simulink model "sim_validate_rint"  (Simulink 3.00)
settings: Solver=ode1  StartTime=starttime  StopTime=endtime  FixedStep=.5  RelTol=1e-3
values from neighbouring files (symbols this model uses):
  pwr_data = -1*pwr_data    [validate_rc.m]    (also in validate_rc_results.m = pwr_data(1:endi); validate_rc_results_2models.m = pwr_data(1:endi))
  t_data = t_data-t_data(1)    [validate_rc.m]    (also in validate_rc_results.m = t_data(1:endi); validate_rc_results_2models.m = t_data(1:endi))
libraries: lib_energy_storage x1
settings Model: LastModifiedBy=vjohnson

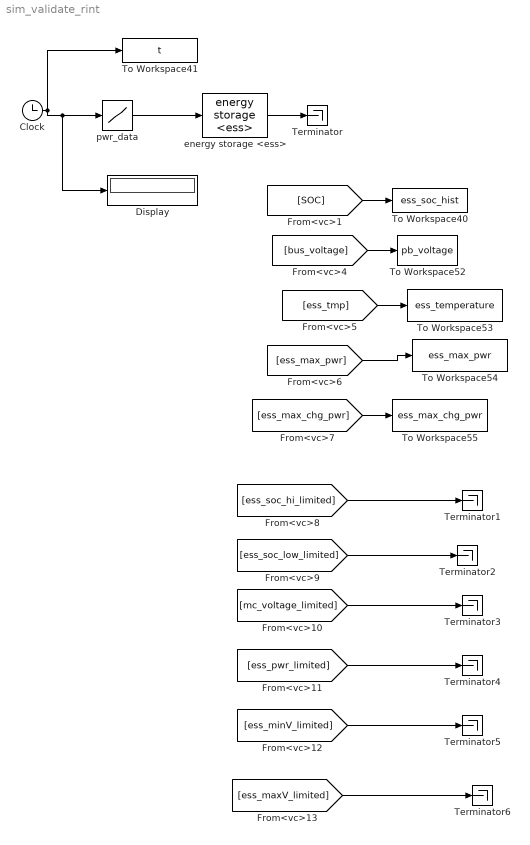
== system sim_validate_rint ==
  Clock : Clock
      settings: DisplayTime=off  Decimation=10
  Display : Display
      settings: Format=short
  Terminator{,1..6} (7 alike) : Terminator
  To Workspace40 : ToWorkspace  VariableName=ess_soc_hist  SampleTime=-1  SaveFormat=Matrix
  To Workspace41 : ToWorkspace  VariableName=t  SampleTime=-1  SaveFormat=Matrix
  To Workspace52 : ToWorkspace  VariableName=pb_voltage  SampleTime=-1  SaveFormat=Matrix
  To Workspace53 : ToWorkspace  VariableName=ess_temperature  SampleTime=-1  SaveFormat=Matrix
  To Workspace54 : ToWorkspace  VariableName=ess_max_pwr  SampleTime=-1  SaveFormat=Matrix
  To Workspace55 : ToWorkspace  VariableName=ess_max_chg_pwr  SampleTime=-1  SaveFormat=Matrix
  energy storage <ess> : lib_energy_storage/energy storage <ess>
  pwr_data : Lookup  InputValues=t_data  OutputValues=pwr_data
  wires:
  pwr_data/1 -> energy storage <ess>/1
  energy storage <ess>/1 -> Terminator/1
  [bus_voltage] -> To Workspace52/1
  [SOC] -> To Workspace40/1
  [ess_tmp] -> To Workspace53/1
  [ess_max_pwr] -> To Workspace54/1
  [ess_max_chg_pwr] -> To Workspace55/1
  Clock/1 -> To Workspace41/1, pwr_data/1, Display/1
  [ess_soc_hi_limited] -> Terminator1/1
  [ess_soc_low_limited] -> Terminator2/1
  [mc_voltage_limited] -> Terminator3/1
  [ess_pwr_limited] -> Terminator4/1
  [ess_minV_limited] -> Terminator5/1
  [ess_maxV_limited] -> Terminator6/1
